simulink model "watertank_compare"  (R2026a)
settings: Solver=VariableStepAuto  StopTime=Tf
PreLoadFcn:
  | Ts = 1; Tf = 100;
InitFcn:
  | Ts = 1; Tf = 100;
StopFcn:
  | plot_comparison
undefined symbols (not defined in the file or in its folder): DiscIntNeverNeededParam
libraries: simulink x3, slpidlib x2
settings Model: Creator=Dharu  LastModifiedBy=Dharu

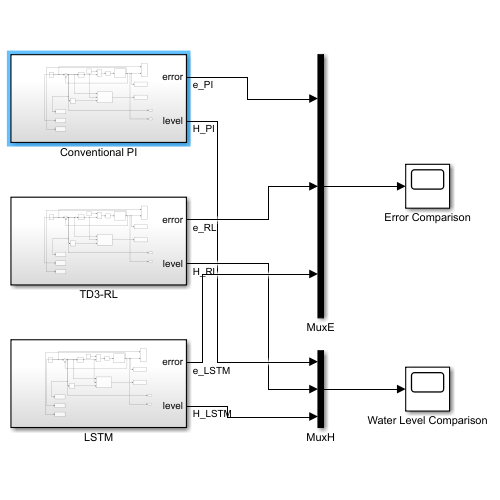
[thumbnail: Simulink's stored preview of the top-level diagram]
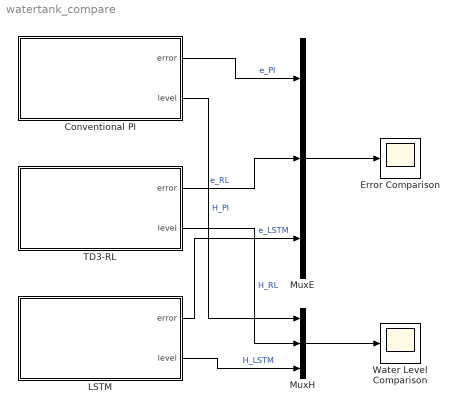
== system watertank_compare ==
  Conventional PI : Subsystem
  Error Comparison : Scope
      settings: Title=Error Comparison  ActiveDisplayYMinimum=-1
  LSTM : Subsystem
  MuxE : Mux  Inputs=3
  MuxH : Mux  Inputs=3
  TD3-RL : Subsystem
  Water Level Comparison : Scope
      settings: Title=Water Level Comparison  ActiveDisplayYMinimum=0  ActiveDisplayYMaximum=12
  wires:
  MuxE/1 -> Error Comparison/1
  MuxH/1 -> Water Level Comparison/1
  Conventional PI/1(error) -> MuxE/1  "e_PI"
  Conventional PI/2(level) -> MuxH/1  "H_PI"
  TD3-RL/1(error) -> MuxE/2  "e_RL"
  TD3-RL/2(level) -> MuxH/2  "H_RL"
  LSTM/1(error) -> MuxE/3  "e_LSTM"
  LSTM/2(level) -> MuxH/3  "H_LSTM"

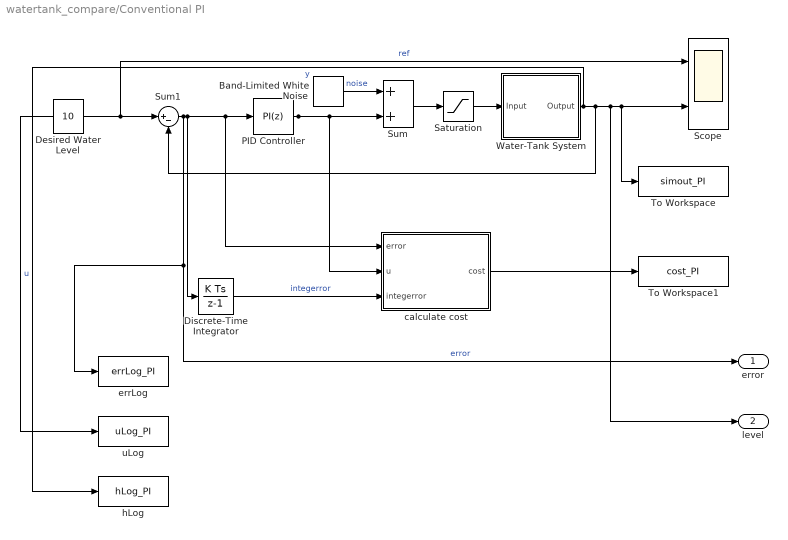
== system watertank_compare/Conventional PI ==
  Band-Limited White Noise : simulink/Sources/Band-Limited White Noise  Cov=0.01  Ts=Ts  seed=1
  Desired Water Level : Constant  Value=10
  Discrete-Time Integrator : DiscreteIntegrator  gainval=1  SampleTime=Ts  LimitOutput=on  UpperSaturationLimit=100  LowerSaturationLimit=-100  ICPrevOutput=DiscIntNeverNeededParam  ICPrevScaledInput=DiscIntNeverNeededParam
  PID Controller : slpidlib/PID Controller  Tag=PID1  Controller=PI  Form=Parallel  TimeDomain=Discrete-time  UseExternalTs=off  SampleTime=Ts  IntegratorMethod=Forward Euler  FilterMethod=Forward Euler  ControllerParametersSource=internal  P=3.437265959  I=0.0357784909  UseKiTs=off  D=-7.525674  UseExternalDerivativeSource=off  N=0.201208  UseFilter=on  TunerSelectOption=Transfer Function Based (PID Tuner App)  ZeroCross=off  InitialConditionSource=internal  InitialConditionForIntegrator=0  InitialConditionForFilter=0  DifferentiatorICPrevScaledInput=0  ExternalReset=none  TrackingMode=off  Kt=1  LimitOutput=off  SatLimitsSource=internal  UpperSaturationLimit=inf  LowerSaturationLimit=-inf  LinearizeAsGain=off  AntiWindupMode=none  Kb=1  LimitIntegrator=off  UpperIntegratorSaturationLimit=inf  LowerIntegratorSaturationLimit=-inf  POutMin=[ ]  POutMax=[ ]  IOutMin=[ ]  IOutMax=[ ]  DOutMin=[ ]  DOutMax=[ ]  NOutMin=[ ]  NOutMax=[ ]  SumOutMin=[ ]  SumOutMax=[ ]  SaturationOutMin=[ ]  SaturationOutMax=[ ]  PParamMin=[ ]  PParamMax=[ ]  IParamMin=[ ]  IParamMax=[ ]  DParamMin=[ ]  DParamMax=[ ]  NParamMin=[ ]  NParamMax=[ ]  KbParamMin=[ ]  KbParamMax=[ ]  KtParamMin=[ ]  KtParamMax=[ ]  KbOutMin=[ ]  KbOutMax=[ ]  KtOutMin=[ ]  KtOutMax=[ ]  IntegratorOutMin=[ ]  IntegratorOutMax=[ ]  FilterOutMin=[ ]  FilterOutMax=[ ]  SumI1OutMin=[ ]  SumI1OutMax=[ ]  SumI2OutMin=[ ]  SumI2OutMax=[ ]  SumI3OutMin=[ ]  SumI3OutMax=[ ]  SumI4OutMin=[]  SumI4OutMax=[]  SumDOutMin=[ ]  SumDOutMax=[ ]  DifferentiatorOutMin=[]  DifferentiatorOutMax=[]  FilterDiffOutCoefMin=[]  FilterDiffOutCoefMax=[]  ReciprocalOutMin=[]  ReciprocalOutMax=[]  SumDenOutMin=[]  SumDenOutMax=[]  SumNumOutMin=[]  SumNumOutMax=[]  DivideOutMin=[]  DivideOutMax=[]  UdiffTsProdOutMin=[]  UdiffTsProdOutMax=[]  NTsProdOutMin=[]  NTsProdOutMax=[]  UintegralTsProdOutMin=[]  UintegralTsProdOutMax=[]  UngainTsProdOutMin=[]  UngainTsProdOutMax=[]  ClampingZeroOutDataTypeStr=Inherit: Inherit via back propagation  ClampingZeroOutMin=[]  ClampingZeroOutMax=[]  FilterDenConstantOutDataTypeStr=Inherit: Inherit via back propagation  FilterDenConstantOutMin=[]  FilterDenConstantOutMax=[]  PCopyOutDataTypeStr=Inherit: Inherit via back propagation  PCopyOutMin=[]  PCopyOutMax=[]  NCopyOutDataTypeStr=Inherit: Inherit via back propagation  NCopyOutMin=[]  NCopyOutMax=[]  IntegratorContinuousStateAttributes=''  IntegratorStateMustResolveToSignalObject=off  IntegratorRTWStateStorageClass=Auto  FilterContinuousStateAttributes=''  FilterStateMustResolveToSignalObject=off  FilterRTWStateStorageClass=Auto  ParallelPVariant=InternalParameters  IdealPVariant=Disabled  IVariant=InternalParameters  DVariant=Disabled  IntegratorVariant=Discrete  SatVariant=Disabled  AWVariant=Passthrough  PCopyVariant=Disabled  TRVariant=Disabled  FdbkBlocksVariant=Forward  IdealPFdbkVariant=Disabled  SatFdbkVariant=Disabled  DerivativeFilterVariant=Disabled  NVariant=Disabled  NCopyVariant=Disabled_SignalSpec  FilterICVariant=Disabled  IntegratorICVariant=InternalICs  ExternalResetVariant=Disabled  TRSumVariant=Passthrough  SumFdbkVariant=Disabled  SumVariant=Sum_PI  TsampFilterVariant=InternalTs  TsampNgainVariant=Passthrough  TsampIntegralVariant=Disabled_SignalSpec  ExternalSaturationOutDataTypeStr=Inherit: Same as second input  DerivativeSourceVariant=Disabled  PreIntVariant=InternalPreInt
  Saturation : Saturate  UpperLimit=12  LowerLimit=0
  Scope : Scope  NumInputPorts=2
      settings: ActiveDisplayYMinimum=-8.8693854504523131  ActiveDisplayYMaximum=18.205080928572428
  Sum : Sum
  Sum1 : Sum  Inputs=|+-  SaturateOnIntegerOverflow=on
  To Workspace : ToWorkspace  VariableName=simout_PI  SaveFormat=Timeseries  SampleTime=-1
  To Workspace1 : ToWorkspace  VariableName=cost_PI  SaveFormat=Timeseries  SampleTime=-1
  Water-Tank System : Subsystem
  calculate cost : Subsystem
  errLog : ToWorkspace  VariableName=errLog_PI  SaveFormat=Timeseries  SampleTime=Ts
  hLog : ToWorkspace  VariableName=hLog_PI  SaveFormat=Timeseries  SampleTime=Ts
  uLog : ToWorkspace  VariableName=uLog_PI  SaveFormat=Timeseries  SampleTime=Ts
  error : Outport
  level : Outport  Port=2
  wires:
  Desired Water Level/1 -> Sum1/1, Scope/1  "ref"
  Sum1/1 -> errLog/1, error/1, PID Controller/1, calculate cost/1(error), Discrete-Time Integrator/1  "error"
  Water-Tank System/1(Output) -> level/1, Scope/2, To Workspace/1, Sum1/2, hLog/1  "y"
  Sum/1 -> Saturation/1
  PID Controller/1 -> uLog/1, Sum/2, calculate cost/2(u)  "u"
  Band-Limited White Noise/1 -> Sum/1  "noise"
  calculate cost/1(cost) -> To Workspace1/1
  Saturation/1 -> Water-Tank System/1(Input)
  Discrete-Time Integrator/1 -> calculate cost/3(integerror)  "integerror"

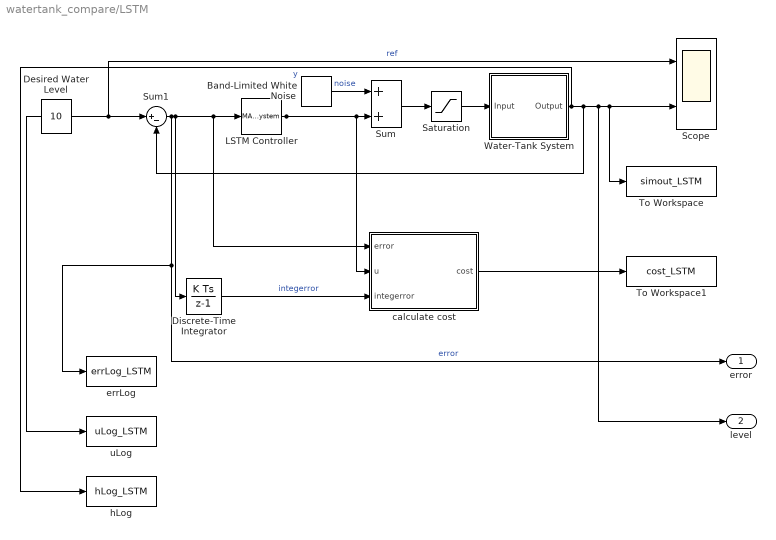
== system watertank_compare/LSTM ==
  Band-Limited White Noise : simulink/Sources/Band-Limited White Noise  Cov=0.01  Ts=Ts  seed=1
  Desired Water Level : Constant  Value=10
  Discrete-Time Integrator : DiscreteIntegrator  gainval=1  SampleTime=Ts  LimitOutput=on  UpperSaturationLimit=100  LowerSaturationLimit=-100  ICPrevOutput=DiscIntNeverNeededParam  ICPrevScaledInput=DiscIntNeverNeededParam
  LSTM Controller : MATLABSystem  System=LSTMController  NetFile=lstmController.mat  Ts=Ts
      mask Type: LSTMController
  Saturation : Saturate  UpperLimit=12  LowerLimit=0
  Scope : Scope  NumInputPorts=2
      settings: ActiveDisplayYMinimum=-8.8693854504523131  ActiveDisplayYMaximum=18.205080928572428  DataLoggingVariableName=ScopeData2
  Sum : Sum
  Sum1 : Sum  Inputs=|+-  SaturateOnIntegerOverflow=on
  To Workspace : ToWorkspace  VariableName=simout_LSTM  SaveFormat=Timeseries  SampleTime=-1
  To Workspace1 : ToWorkspace  VariableName=cost_LSTM  SaveFormat=Timeseries  SampleTime=-1
  Water-Tank System : Subsystem
  calculate cost : Subsystem
  errLog : ToWorkspace  VariableName=errLog_LSTM  SaveFormat=Timeseries  SampleTime=Ts
  hLog : ToWorkspace  VariableName=hLog_LSTM  SaveFormat=Timeseries  SampleTime=Ts
  uLog : ToWorkspace  VariableName=uLog_LSTM  SaveFormat=Timeseries  SampleTime=Ts
  error : Outport
  level : Outport  Port=2
  wires:
  Desired Water Level/1 -> Sum1/1, Scope/1  "ref"
  Sum1/1 -> errLog/1, error/1, LSTM Controller/1, calculate cost/1(error), Discrete-Time Integrator/1  "error"
  Water-Tank System/1(Output) -> level/1, Scope/2, To Workspace/1, Sum1/2, hLog/1  "y"
  Sum/1 -> Saturation/1
  Band-Limited White Noise/1 -> Sum/1  "noise"
  calculate cost/1(cost) -> To Workspace1/1
  Saturation/1 -> Water-Tank System/1(Input)
  Discrete-Time Integrator/1 -> calculate cost/3(integerror)  "integerror"
  LSTM Controller/1 -> Sum/2, calculate cost/2(u), uLog/1

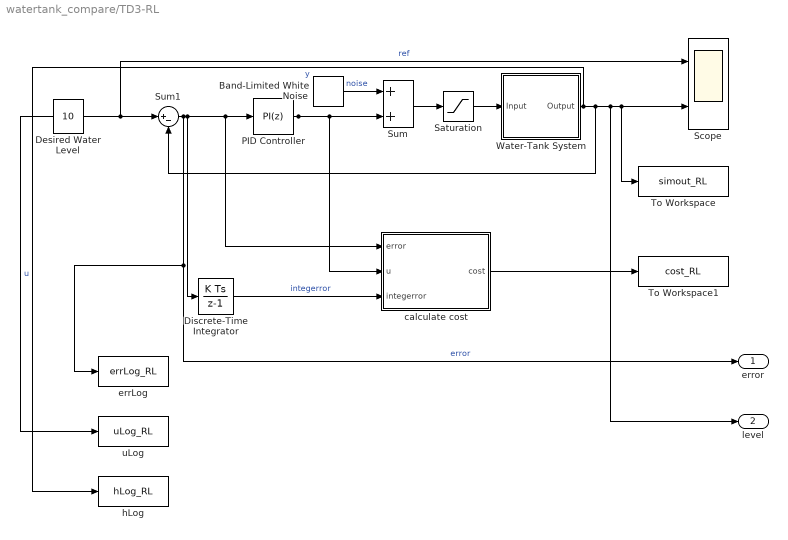
== system watertank_compare/TD3-RL ==
  Band-Limited White Noise : simulink/Sources/Band-Limited White Noise  Cov=0.01  Ts=Ts  seed=1
  Desired Water Level : Constant  Value=10
  Discrete-Time Integrator : DiscreteIntegrator  gainval=1  SampleTime=Ts  LimitOutput=on  UpperSaturationLimit=100  LowerSaturationLimit=-100  ICPrevOutput=DiscIntNeverNeededParam  ICPrevScaledInput=DiscIntNeverNeededParam
  PID Controller : slpidlib/PID Controller  Tag=PID1  Controller=PI  Form=Parallel  TimeDomain=Discrete-time  UseExternalTs=off  SampleTime=Ts  IntegratorMethod=Forward Euler  FilterMethod=Forward Euler  ControllerParametersSource=internal  P=3.808981657  I=0.1130104288  UseKiTs=off  D=-7.525674  UseExternalDerivativeSource=off  N=0.201208  UseFilter=on  TunerSelectOption=Transfer Function Based (PID Tuner App)  ZeroCross=off  InitialConditionSource=internal  InitialConditionForIntegrator=0  InitialConditionForFilter=0  DifferentiatorICPrevScaledInput=0  ExternalReset=none  TrackingMode=off  Kt=1  LimitOutput=off  SatLimitsSource=internal  UpperSaturationLimit=inf  LowerSaturationLimit=-inf  LinearizeAsGain=off  AntiWindupMode=none  Kb=1  LimitIntegrator=off  UpperIntegratorSaturationLimit=inf  LowerIntegratorSaturationLimit=-inf  POutMin=[ ]  POutMax=[ ]  IOutMin=[ ]  IOutMax=[ ]  DOutMin=[ ]  DOutMax=[ ]  NOutMin=[ ]  NOutMax=[ ]  SumOutMin=[ ]  SumOutMax=[ ]  SaturationOutMin=[ ]  SaturationOutMax=[ ]  PParamMin=[ ]  PParamMax=[ ]  IParamMin=[ ]  IParamMax=[ ]  DParamMin=[ ]  DParamMax=[ ]  NParamMin=[ ]  NParamMax=[ ]  KbParamMin=[ ]  KbParamMax=[ ]  KtParamMin=[ ]  KtParamMax=[ ]  KbOutMin=[ ]  KbOutMax=[ ]  KtOutMin=[ ]  KtOutMax=[ ]  IntegratorOutMin=[ ]  IntegratorOutMax=[ ]  FilterOutMin=[ ]  FilterOutMax=[ ]  SumI1OutMin=[ ]  SumI1OutMax=[ ]  SumI2OutMin=[ ]  SumI2OutMax=[ ]  SumI3OutMin=[ ]  SumI3OutMax=[ ]  SumI4OutMin=[]  SumI4OutMax=[]  SumDOutMin=[ ]  SumDOutMax=[ ]  DifferentiatorOutMin=[]  DifferentiatorOutMax=[]  FilterDiffOutCoefMin=[]  FilterDiffOutCoefMax=[]  ReciprocalOutMin=[]  ReciprocalOutMax=[]  SumDenOutMin=[]  SumDenOutMax=[]  SumNumOutMin=[]  SumNumOutMax=[]  DivideOutMin=[]  DivideOutMax=[]  UdiffTsProdOutMin=[]  UdiffTsProdOutMax=[]  NTsProdOutMin=[]  NTsProdOutMax=[]  UintegralTsProdOutMin=[]  UintegralTsProdOutMax=[]  UngainTsProdOutMin=[]  UngainTsProdOutMax=[]  ClampingZeroOutDataTypeStr=Inherit: Inherit via back propagation  ClampingZeroOutMin=[]  ClampingZeroOutMax=[]  FilterDenConstantOutDataTypeStr=Inherit: Inherit via back propagation  FilterDenConstantOutMin=[]  FilterDenConstantOutMax=[]  PCopyOutDataTypeStr=Inherit: Inherit via back propagation  PCopyOutMin=[]  PCopyOutMax=[]  NCopyOutDataTypeStr=Inherit: Inherit via back propagation  NCopyOutMin=[]  NCopyOutMax=[]  IntegratorContinuousStateAttributes=''  IntegratorStateMustResolveToSignalObject=off  IntegratorRTWStateStorageClass=Auto  FilterContinuousStateAttributes=''  FilterStateMustResolveToSignalObject=off  FilterRTWStateStorageClass=Auto  ParallelPVariant=InternalParameters  IdealPVariant=Disabled  IVariant=InternalParameters  DVariant=Disabled  IntegratorVariant=Discrete  SatVariant=Disabled  AWVariant=Passthrough  PCopyVariant=Disabled  TRVariant=Disabled  FdbkBlocksVariant=Forward  IdealPFdbkVariant=Disabled  SatFdbkVariant=Disabled  DerivativeFilterVariant=Disabled  NVariant=Disabled  NCopyVariant=Disabled_SignalSpec  FilterICVariant=Disabled  IntegratorICVariant=InternalICs  ExternalResetVariant=Disabled  TRSumVariant=Passthrough  SumFdbkVariant=Disabled  SumVariant=Sum_PI  TsampFilterVariant=InternalTs  TsampNgainVariant=Passthrough  TsampIntegralVariant=Disabled_SignalSpec  ExternalSaturationOutDataTypeStr=Inherit: Same as second input  DerivativeSourceVariant=Disabled  PreIntVariant=InternalPreInt
  Saturation : Saturate  UpperLimit=12  LowerLimit=0
  Scope : Scope  NumInputPorts=2
      settings: ActiveDisplayYMinimum=-8.8693854504523131  ActiveDisplayYMaximum=18.205080928572428
  Sum : Sum
  Sum1 : Sum  Inputs=|+-  SaturateOnIntegerOverflow=on
  To Workspace : ToWorkspace  VariableName=simout_RL  SaveFormat=Timeseries  SampleTime=-1
  To Workspace1 : ToWorkspace  VariableName=cost_RL  SaveFormat=Timeseries  SampleTime=-1
  Water-Tank System : Subsystem
  calculate cost : Subsystem
  errLog : ToWorkspace  VariableName=errLog_RL  SaveFormat=Timeseries  SampleTime=Ts
  hLog : ToWorkspace  VariableName=hLog_RL  SaveFormat=Timeseries  SampleTime=Ts
  uLog : ToWorkspace  VariableName=uLog_RL  SaveFormat=Timeseries  SampleTime=Ts
  error : Outport
  level : Outport  Port=2
  wires:
  Desired Water Level/1 -> Sum1/1, Scope/1  "ref"
  Sum1/1 -> errLog/1, error/1, PID Controller/1, calculate cost/1(error), Discrete-Time Integrator/1  "error"
  Water-Tank System/1(Output) -> level/1, Scope/2, To Workspace/1, Sum1/2, hLog/1  "y"
  Sum/1 -> Saturation/1
  PID Controller/1 -> uLog/1, Sum/2, calculate cost/2(u)  "u"
  Band-Limited White Noise/1 -> Sum/1  "noise"
  calculate cost/1(cost) -> To Workspace1/1
  Saturation/1 -> Water-Tank System/1(Input)
  Discrete-Time Integrator/1 -> calculate cost/3(integerror)  "integerror"

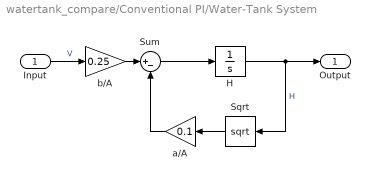
== system watertank_compare/Conventional PI/Water-Tank System ==
  Input : Inport
  H : Integrator  InitialCondition=1  LimitOutput=on  LowerSaturationLimit=0
  Sqrt : Sqrt  OutputSignalType=real
  Sum : Sum  Inputs=|+-  SaturateOnIntegerOverflow=on
  a/A : Gain  Gain=0.1  SaturateOnIntegerOverflow=on  OutDataTypeStr=Inherit: Same as input  ParamDataTypeStr=Inherit: Same as input
  b/A : Gain  Gain=0.25  SaturateOnIntegerOverflow=on  OutDataTypeStr=Inherit: Same as input  ParamDataTypeStr=Inherit: Same as input
  Output : Outport  VectorParamsAs1DForOutWhenUnconnected=off
  wires:
  Input/1 -> b/A/1  "V"
  a/A/1 -> Sum/2
  Sqrt/1 -> a/A/1
  H/1 -> Output/1, Sqrt/1  "H"
  Sum/1 -> H/1
  b/A/1 -> Sum/1

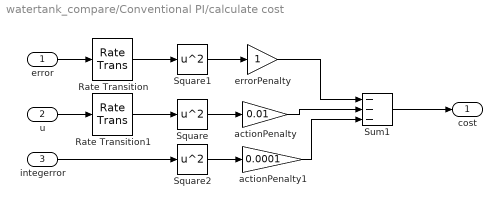
== system watertank_compare/Conventional PI/calculate cost ==
  error : Inport
  u : Inport  Port=2
  integerror : Inport  Port=3
  Rate Transition : RateTransition  OutPortSampleTime=Ts
  Rate Transition1 : RateTransition  OutPortSampleTime=Ts
  Square : Math  Operator=square
  Square1 : Math  Operator=square
  Square2 : Math  Operator=square
  Sum1 : Sum  Inputs=---  OutDataTypeStr=double
  actionPenalty : Gain  Gain=0.01
  actionPenalty1 : Gain  Gain=0.0001
  errorPenalty : Gain
  cost : Outport  VectorParamsAs1DForOutWhenUnconnected=off
  wires:
  Square2/1 -> actionPenalty1/1
  actionPenalty1/1 -> Sum1/3
  integerror/1 -> Square2/1
  Rate Transition1/1 -> Square/1
  Rate Transition/1 -> Square1/1
  Sum1/1 -> cost/1
  error/1 -> Rate Transition/1
  u/1 -> Rate Transition1/1
  Square/1 -> actionPenalty/1
  actionPenalty/1 -> Sum1/2
  errorPenalty/1 -> Sum1/1
  Square1/1 -> errorPenalty/1

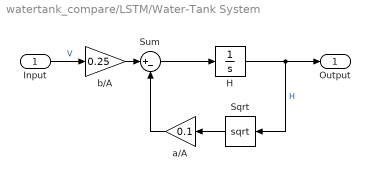
== system watertank_compare/LSTM/Water-Tank System ==
  Input : Inport
  H : Integrator  InitialCondition=1  LimitOutput=on  LowerSaturationLimit=0
  Sqrt : Sqrt  OutputSignalType=real
  Sum : Sum  Inputs=|+-  SaturateOnIntegerOverflow=on
  a/A : Gain  Gain=0.1  SaturateOnIntegerOverflow=on  OutDataTypeStr=Inherit: Same as input  ParamDataTypeStr=Inherit: Same as input
  b/A : Gain  Gain=0.25  SaturateOnIntegerOverflow=on  OutDataTypeStr=Inherit: Same as input  ParamDataTypeStr=Inherit: Same as input
  Output : Outport  VectorParamsAs1DForOutWhenUnconnected=off
  wires:
  Input/1 -> b/A/1  "V"
  a/A/1 -> Sum/2
  Sqrt/1 -> a/A/1
  H/1 -> Output/1, Sqrt/1  "H"
  Sum/1 -> H/1
  b/A/1 -> Sum/1

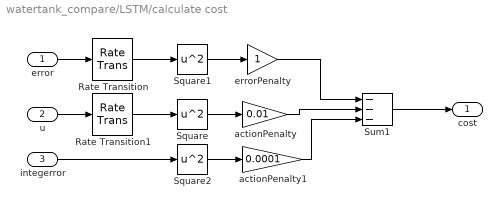
== system watertank_compare/LSTM/calculate cost ==
  error : Inport
  u : Inport  Port=2
  integerror : Inport  Port=3
  Rate Transition : RateTransition  OutPortSampleTime=Ts
  Rate Transition1 : RateTransition  OutPortSampleTime=Ts
  Square : Math  Operator=square
  Square1 : Math  Operator=square
  Square2 : Math  Operator=square
  Sum1 : Sum  Inputs=---  OutDataTypeStr=double
  actionPenalty : Gain  Gain=0.01
  actionPenalty1 : Gain  Gain=0.0001
  errorPenalty : Gain
  cost : Outport  VectorParamsAs1DForOutWhenUnconnected=off
  wires:
  Square2/1 -> actionPenalty1/1
  actionPenalty1/1 -> Sum1/3
  integerror/1 -> Square2/1
  Rate Transition1/1 -> Square/1
  Rate Transition/1 -> Square1/1
  Sum1/1 -> cost/1
  error/1 -> Rate Transition/1
  u/1 -> Rate Transition1/1
  Square/1 -> actionPenalty/1
  actionPenalty/1 -> Sum1/2
  errorPenalty/1 -> Sum1/1
  Square1/1 -> errorPenalty/1

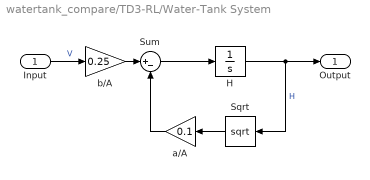
== system watertank_compare/TD3-RL/Water-Tank System ==
  Input : Inport
  H : Integrator  InitialCondition=1  LimitOutput=on  LowerSaturationLimit=0
  Sqrt : Sqrt  OutputSignalType=real
  Sum : Sum  Inputs=|+-  SaturateOnIntegerOverflow=on
  a/A : Gain  Gain=0.1  SaturateOnIntegerOverflow=on  OutDataTypeStr=Inherit: Same as input  ParamDataTypeStr=Inherit: Same as input
  b/A : Gain  Gain=0.25  SaturateOnIntegerOverflow=on  OutDataTypeStr=Inherit: Same as input  ParamDataTypeStr=Inherit: Same as input
  Output : Outport  VectorParamsAs1DForOutWhenUnconnected=off
  wires:
  Input/1 -> b/A/1  "V"
  a/A/1 -> Sum/2
  Sqrt/1 -> a/A/1
  H/1 -> Output/1, Sqrt/1  "H"
  Sum/1 -> H/1
  b/A/1 -> Sum/1

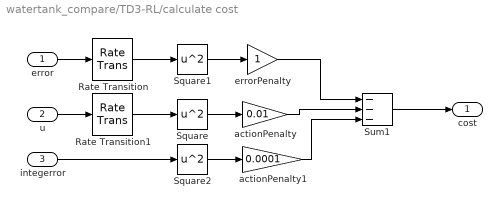
== system watertank_compare/TD3-RL/calculate cost ==
  error : Inport
  u : Inport  Port=2
  integerror : Inport  Port=3
  Rate Transition : RateTransition  OutPortSampleTime=Ts
  Rate Transition1 : RateTransition  OutPortSampleTime=Ts
  Square : Math  Operator=square
  Square1 : Math  Operator=square
  Square2 : Math  Operator=square
  Sum1 : Sum  Inputs=---  OutDataTypeStr=double
  actionPenalty : Gain  Gain=0.01
  actionPenalty1 : Gain  Gain=0.0001
  errorPenalty : Gain
  cost : Outport  VectorParamsAs1DForOutWhenUnconnected=off
  wires:
  Square2/1 -> actionPenalty1/1
  actionPenalty1/1 -> Sum1/3
  integerror/1 -> Square2/1
  Rate Transition1/1 -> Square/1
  Rate Transition/1 -> Square1/1
  Sum1/1 -> cost/1
  error/1 -> Rate Transition/1
  u/1 -> Rate Transition1/1
  Square/1 -> actionPenalty/1
  actionPenalty/1 -> Sum1/2
  errorPenalty/1 -> Sum1/1
  Square1/1 -> errorPenalty/1
